simulink model "OpAmpCircuits2"  (R2021b)
settings: Solver=VariableStepAuto  StartTime=0.0  StopTime=inf  MaxStep=1e-5  RelTol=1e-3
libraries: fl_lib x55, nesl_utility x20, simulink x1
settings Model: PacingRate=0.010000  Creator=Work  LastModifiedBy=Work

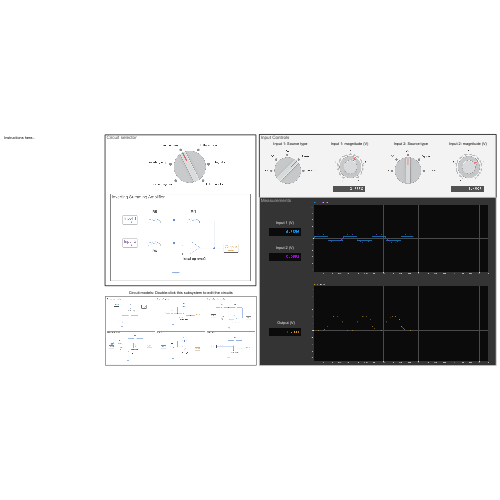
[thumbnail: Simulink's stored preview of the top-level diagram]
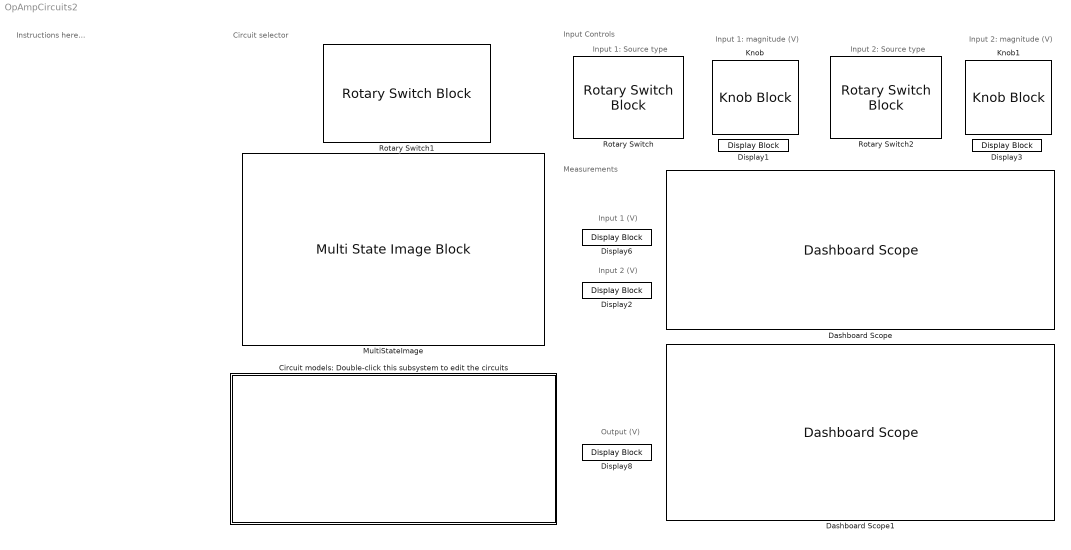
== system OpAmpCircuits2 ==
  note: Instructions here...
  note: Circuit selector
  note: Input 1: magnitude (V)
  note: Input 1: Source type
  note: Input Controls
  note: Measurements
  note: Input 1 (V)
  note: Output (V)
  note: Input 2 (V)
  note: Input 2: Source type
  note: Input 2: magnitude (V)
  Circuit models: Double-click this subsystem to edit the circuits : Subsystem
      mask Display: image('opampcircuits.png')
  Dashboard Scope : DashboardScope  TimeSpan=0.10000000000000001  Ymin=-11  Ymax=11  ScaleAtStop=off
  Dashboard Scope1 : DashboardScope  TimeSpan=0.10000000000000001  Ymin=-11  Ymax=11  ScaleAtStop=off
  Display{1..3,6,8} (5 alike) : DisplayBlock  LabelPosition=Hide  Format=Custom  Alignment=Right  Transparency=1  FormatString=%0.4f
  Knob : KnobBlock  LabelPosition=Hide  ScaleMin=-4  ScaleMax=4  TickInterval=2
  Knob1 : KnobBlock  LabelPosition=Hide  ScaleMin=-4  ScaleMax=4  TickInterval=2
  MultiStateImage : MultiStateImageBlock  LabelPosition=Hide
  Rotary Switch : RotarySwitchBlock  LabelPosition=Hide
      settings: Values={{'Off', 'DC', 'AC', 'Square', 'Triangle'}, [0 1 2 3 4]}
  Rotary Switch1 : RotarySwitchBlock  LabelPosition=Hide
      settings: Values={{'Noninverting amp', 'Inverting amp', 'Summing amp', 'Difference amp', 'Integrator', 'Differentiator'}, [1 2 3 4 5 6]}
  Rotary Switch2 : RotarySwitchBlock  LabelPosition=Hide
      settings: Values={{'Off', 'DC', 'AC', 'Square', 'Triangle'}, [0 1 2 3 4]}

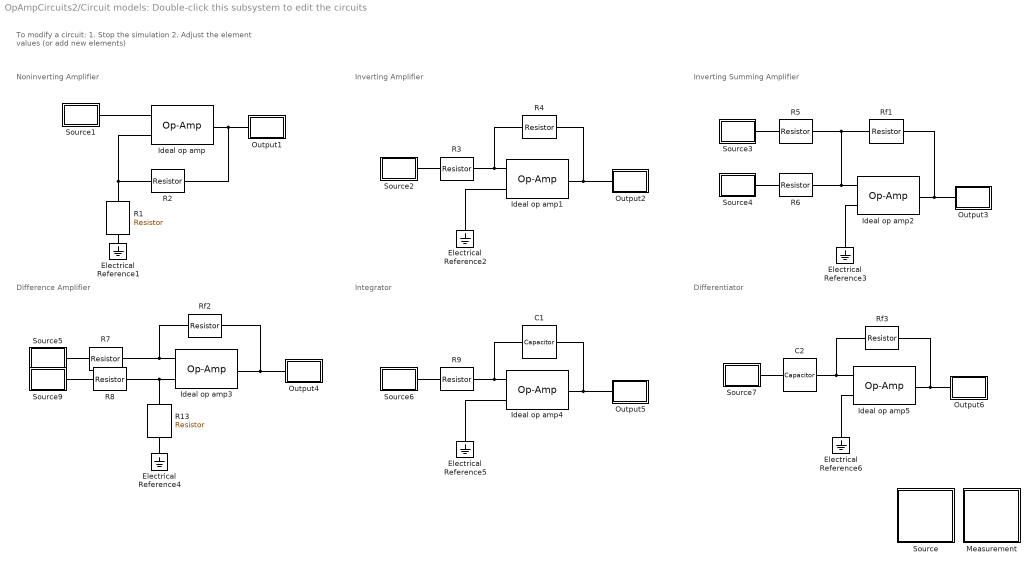
== system OpAmpCircuits2/Circuit models: Double-click this subsystem to edit the circuits ==
  note: To modify a circuit:
      |    1. Stop the simulation
      |    2. Adjust the element values (or add new elements)
  note: Differentiator
  note: Integrator
  note: Difference Amplifier
  note: Inverting Summing Amplifier
  note: Inverting Amplifier
  note: Noninverting Amplifier
  C1 : fl_lib/Electrical/Electrical Elements/Capacitor  c=1 uF  r=1e-6 Ohm  g=0 1/Ohm  i_specify=off  i_priority=None  i=0 A  i_nominal_specify=off  i_nominal_unit=A  i_nominal_value=1  v_specify=off  v_priority=None  v=0 V  v_nominal_specify=off  v_nominal_unit=V  v_nominal_value=1  vc_specify=off  vc_priority=High  vc=0 V  vc_nominal_specify=off  vc_nominal_unit=V  vc_nominal_value=1
      settings: AttributesFormatString=%<c> %<c_unit>
  C2 : fl_lib/Electrical/Electrical Elements/Capacitor  c=1 uF  r=1e-6 Ohm  g=0 1/Ohm  i_specify=off  i_priority=None  i=0 A  i_nominal_specify=off  i_nominal_unit=A  i_nominal_value=1  v_specify=off  v_priority=None  v=0 V  v_nominal_specify=off  v_nominal_unit=V  v_nominal_value=1  vc_specify=off  vc_priority=High  vc=0 V  vc_nominal_specify=off  vc_nominal_unit=V  vc_nominal_value=1
      settings: AttributesFormatString=%<c> %<c_unit>
  Electrical Reference{1..6} (6 alike) : fl_lib/Electrical/Electrical Elements/Electrical Reference
  Ideal op amp{,1..5} (6 alike) : fl_lib/Electrical/Electrical Elements/Op-Amp  outI_specify=off  outI_priority=None  outI=0 A  outI_nominal_specify=off  outI_nominal_unit=A  outI_nominal_value=1
  Measurement : Subsystem
  Output1 : Subsystem
      mask Display: image("output.png")
  Output2 : Subsystem
      mask Display: image("output.png")
  Output3 : Subsystem
      mask Display: image("output.png")
  Output4 : Subsystem
      mask Display: image("output.png")
  Output5 : Subsystem
      mask Display: image("output.png")
  Output6 : Subsystem
      mask Display: image("output.png")
  R{1..3,5..8,13} (8 alike) : fl_lib/Electrical/Electrical Elements/Resistor  R=1 kOhm  i_specify=off  i_priority=None  i=0 A  i_nominal_specify=off  i_nominal_unit=A  i_nominal_value=1  v_specify=off  v_priority=None  v=0 V  v_nominal_specify=off  v_nominal_unit=V  v_nominal_value=1
      settings: AttributesFormatString=%<R> %<R_unit>
  R4 : fl_lib/Electrical/Electrical Elements/Resistor  R=2 kOhm  i_specify=off  i_priority=None  i=0 A  i_nominal_specify=off  i_nominal_unit=A  i_nominal_value=1  v_specify=off  v_priority=None  v=0 V  v_nominal_specify=off  v_nominal_unit=V  v_nominal_value=1
      settings: AttributesFormatString=%<R> %<R_unit>
  R9 : fl_lib/Electrical/Electrical Elements/Resistor  R=2 kOhm  i_specify=off  i_priority=None  i=0 A  i_nominal_specify=off  i_nominal_unit=A  i_nominal_value=1  v_specify=off  v_priority=None  v=0 V  v_nominal_specify=off  v_nominal_unit=V  v_nominal_value=1
      settings: AttributesFormatString=%<R> %<R_unit>
  Rf1 : fl_lib/Electrical/Electrical Elements/Resistor  R=1 kOhm  i_specify=off  i_priority=None  i=0 A  i_nominal_specify=off  i_nominal_unit=A  i_nominal_value=1  v_specify=off  v_priority=None  v=0 V  v_nominal_specify=off  v_nominal_unit=V  v_nominal_value=1
      settings: AttributesFormatString=%<R> %<R_unit>
  Rf2 : fl_lib/Electrical/Electrical Elements/Resistor  R=1 kOhm  i_specify=off  i_priority=None  i=0 A  i_nominal_specify=off  i_nominal_unit=A  i_nominal_value=1  v_specify=off  v_priority=None  v=0 V  v_nominal_specify=off  v_nominal_unit=V  v_nominal_value=1
      settings: AttributesFormatString=%<R> %<R_unit>
  Rf3 : fl_lib/Electrical/Electrical Elements/Resistor  R=10 kOhm  i_specify=off  i_priority=None  i=0 A  i_nominal_specify=off  i_nominal_unit=A  i_nominal_value=1  v_specify=off  v_priority=None  v=0 V  v_nominal_specify=off  v_nominal_unit=V  v_nominal_value=1
      settings: AttributesFormatString=%<R> %<R_unit>
  Source : Subsystem
  Source1 : Subsystem
      mask Display: image("input1.png")
  Source2 : Subsystem
      mask Display: image("input1.png")
  Source3 : Subsystem
      mask Display: image("input1.png")
  Source4 : Subsystem
      mask Display: image("input2.png")
  Source5 : Subsystem
      mask Display: image("input1.png")
  Source6 : Subsystem
      mask Display: image("input1.png")
  Source7 : Subsystem
      mask Display: image("input1.png")
  Source9 : Subsystem
      mask Display: image("input2.png")
  connections:
  Ideal op amp5/LConn1 -- Electrical Reference6/LConn1
  Ideal op amp1/RConn1 -- Output2/LConn1 -- R4/LConn1
  R7/RConn1 -- Source5/RConn1
  C2/LConn1 -- Source7/RConn1
  Ideal op amp3/LConn2 -- Rf2/RConn1 -- R7/LConn1
  R8/RConn1 -- Source9/RConn1
  R6/RConn1 -- Source4/RConn1
  Source6/RConn1 -- R9/RConn1
  Ideal op amp4/RConn1 -- C1/RConn1 -- Output5/LConn1
  Output4/LConn1 -- Ideal op amp3/RConn1 -- Rf2/LConn1
  R2/RConn1 -- Ideal op amp/LConn2 -- R1/LConn1
  Ideal op amp/RConn1 -- Output1/LConn1 -- R2/LConn1
  Ideal op amp4/LConn1 -- Electrical Reference5/LConn1
  Source3/RConn1 -- R5/RConn1
  R13/RConn1 -- Electrical Reference4/LConn1
  Ideal op amp2/LConn1 -- Electrical Reference3/LConn1
  Ideal op amp5/LConn2 -- C2/RConn1 -- Rf3/RConn1
  Ideal op amp2/RConn1 -- Output3/LConn1 -- Rf1/LConn1
  Ideal op amp4/LConn2 -- C1/LConn1 -- R9/LConn1
  Ideal op amp1/LConn2 -- R3/LConn1 -- R4/RConn1
  Rf3/LConn1 -- Ideal op amp5/RConn1 -- Output6/LConn1
  Source2/RConn1 -- R3/RConn1
  R1/RConn1 -- Electrical Reference1/LConn1
  Ideal op amp1/LConn1 -- Electrical Reference2/LConn1
  Ideal op amp2/LConn2 -- R6/LConn1 -- R5/LConn1 -- Rf1/RConn1
  R8/LConn1 -- R13/LConn1 -- Ideal op amp3/LConn1
  Ideal op amp/LConn1 -- Source1/RConn1

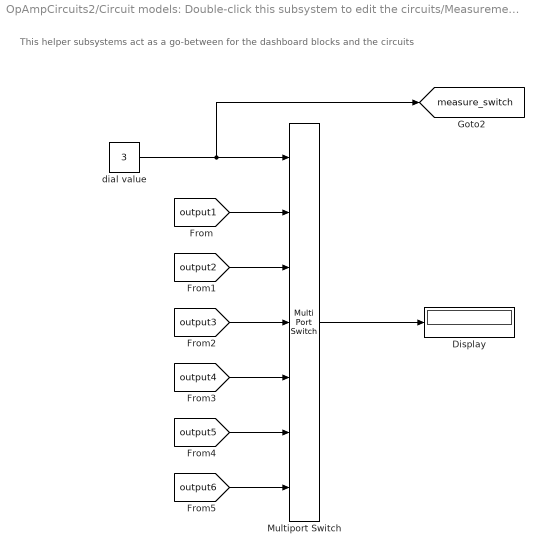
== system OpAmpCircuits2/Circuit models: Double-click this subsystem to edit the circuits/Measurement ==
  note: This helper subsystems act as a go-between for the dashboard blocks and the circuits
  Display : Display
  Multiport Switch : MultiPortSwitch  Inputs=6
  dial value : Constant  Value=3
  tag scope: measure_switch=global
  wires:
  [output1] -> Multiport Switch/2
  [output2] -> Multiport Switch/3
  [output3] -> Multiport Switch/4
  Multiport Switch/1 -> Display/1
  [output4] -> Multiport Switch/5
  [output5] -> Multiport Switch/6
  [output6] -> Multiport Switch/7
  dial value/1 -> [measure_switch], Multiport Switch/1

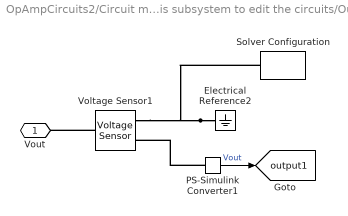
== system OpAmpCircuits2/Circuit models: Double-click this subsystem to edit the circuits/Output1 ==
  Electrical Reference2 : fl_lib/Electrical/Electrical Elements/Electrical Reference
  PS-Simulink Converter1 : nesl_utility/PS-Simulink Converter  PhysicalDomain=network_engine_domain  SubClassName=ps_output  LeftPortType=input  RightPortType=output  PseudoPeriodic=off  Frequencies=[]  Unit=inherit  AffineConversion=off
      settings: SourceProductBaseCode=PW,SS
  Solver Configuration : nesl_utility/Solver Configuration  PhysicalDomain=network_engine_domain  SubClassName=solver  LeftPortType=input  RightPortType=generic  Tones=[]  Harmonics=[]  SimulateNoise=off  Profile=off  UseLocalSampling=off  EnableSwitchedLinearOptims=on  FrequencyDomain=off  UseCCode=off  RelTol=0.001  AbsTol=1e-06  MinStep=1e-09  ToWorkspace=off  RevertToSquareIcSolve=off  NumHomotopyIterations=100  PhasorMode=off  PhasorModeNumHarmonics=1  DoDC=off  ResidualTolerance=1e-09  UseLocalSolver=off  LocalSolverChoice=NE_BACKWARD_EULER_ADVANCER  LocalSolverSampleTime=0.001  DoFixedCost=off  MaxNonlinIter=3  MaxModeIter=2  ComputeImpulses=off  ImpulseIterations=2  LinearAlgebra=auto  EquationFormulation=NE_TIME_EF  DelaysMemoryBudget=1024  AutomaticFiltering=on  FilteringTimeConstant=0.001  PartitionStorageMethod=AS_NEEDED  PartitionMemoryBudget=1024  PartitionMethod=ROBUST
      settings: SourceProductBaseCode=PW,SS
  Voltage Sensor1 : fl_lib/Electrical/Electrical Sensors/Voltage Sensor
  Vout : PMIOPort  Side=Left
  tag scope: output1=global
  wires:
  PS-Simulink Converter1/1 -> [output1]  "Vout"
  connections:
  Voltage Sensor1/LConn1 -- Vout/RConn1
  Electrical Reference2/LConn1 -- Voltage Sensor1/RConn2 -- Solver Configuration/RConn1
  PS-Simulink Converter1/LConn1 -- Voltage Sensor1/RConn1

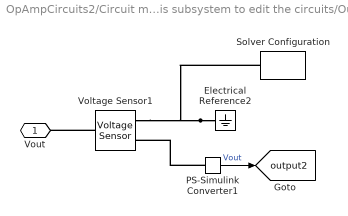
== system OpAmpCircuits2/Circuit models: Double-click this subsystem to edit the circuits/Output2 ==
  Electrical Reference2 : fl_lib/Electrical/Electrical Elements/Electrical Reference
  PS-Simulink Converter1 : nesl_utility/PS-Simulink Converter  PhysicalDomain=network_engine_domain  SubClassName=ps_output  LeftPortType=input  RightPortType=output  PseudoPeriodic=off  Frequencies=[]  Unit=inherit  AffineConversion=off
      settings: SourceProductBaseCode=PW,SS
  Solver Configuration : nesl_utility/Solver Configuration  PhysicalDomain=network_engine_domain  SubClassName=solver  LeftPortType=input  RightPortType=generic  Tones=[]  Harmonics=[]  SimulateNoise=off  Profile=off  UseLocalSampling=off  EnableSwitchedLinearOptims=on  FrequencyDomain=off  UseCCode=off  RelTol=0.001  AbsTol=1e-06  MinStep=1e-09  ToWorkspace=off  RevertToSquareIcSolve=off  NumHomotopyIterations=100  PhasorMode=off  PhasorModeNumHarmonics=1  DoDC=off  ResidualTolerance=1e-09  UseLocalSolver=off  LocalSolverChoice=NE_BACKWARD_EULER_ADVANCER  LocalSolverSampleTime=0.001  DoFixedCost=off  MaxNonlinIter=3  MaxModeIter=2  ComputeImpulses=off  ImpulseIterations=2  LinearAlgebra=auto  EquationFormulation=NE_TIME_EF  DelaysMemoryBudget=1024  AutomaticFiltering=on  FilteringTimeConstant=0.001  PartitionStorageMethod=AS_NEEDED  PartitionMemoryBudget=1024  PartitionMethod=ROBUST
      settings: SourceProductBaseCode=PW,SS
  Voltage Sensor1 : fl_lib/Electrical/Electrical Sensors/Voltage Sensor
  Vout : PMIOPort  Side=Left
  tag scope: output2=global
  wires:
  PS-Simulink Converter1/1 -> [output2]  "Vout"
  connections:
  Voltage Sensor1/LConn1 -- Vout/RConn1
  Electrical Reference2/LConn1 -- Voltage Sensor1/RConn2 -- Solver Configuration/RConn1
  PS-Simulink Converter1/LConn1 -- Voltage Sensor1/RConn1

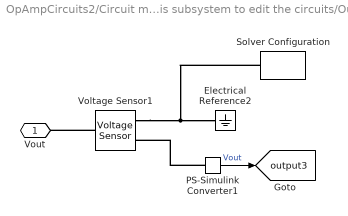
== system OpAmpCircuits2/Circuit models: Double-click this subsystem to edit the circuits/Output3 ==
  Electrical Reference2 : fl_lib/Electrical/Electrical Elements/Electrical Reference
  PS-Simulink Converter1 : nesl_utility/PS-Simulink Converter  PhysicalDomain=network_engine_domain  SubClassName=ps_output  LeftPortType=input  RightPortType=output  PseudoPeriodic=off  Frequencies=[]  Unit=inherit  AffineConversion=off
      settings: SourceProductBaseCode=PW,SS
  Solver Configuration : nesl_utility/Solver Configuration  PhysicalDomain=network_engine_domain  SubClassName=solver  LeftPortType=input  RightPortType=generic  Tones=[]  Harmonics=[]  SimulateNoise=off  Profile=off  UseLocalSampling=off  EnableSwitchedLinearOptims=on  FrequencyDomain=off  UseCCode=off  RelTol=0.001  AbsTol=1e-06  MinStep=1e-09  ToWorkspace=off  RevertToSquareIcSolve=off  NumHomotopyIterations=100  PhasorMode=off  PhasorModeNumHarmonics=1  DoDC=off  ResidualTolerance=1e-09  UseLocalSolver=off  LocalSolverChoice=NE_BACKWARD_EULER_ADVANCER  LocalSolverSampleTime=0.001  DoFixedCost=off  MaxNonlinIter=3  MaxModeIter=2  ComputeImpulses=off  ImpulseIterations=2  LinearAlgebra=auto  EquationFormulation=NE_TIME_EF  DelaysMemoryBudget=1024  AutomaticFiltering=on  FilteringTimeConstant=0.001  PartitionStorageMethod=AS_NEEDED  PartitionMemoryBudget=1024  PartitionMethod=ROBUST
      settings: SourceProductBaseCode=PW,SS
  Voltage Sensor1 : fl_lib/Electrical/Electrical Sensors/Voltage Sensor
  Vout : PMIOPort  Side=Left
  tag scope: output3=global
  wires:
  PS-Simulink Converter1/1 -> [output3]  "Vout"
  connections:
  Voltage Sensor1/LConn1 -- Vout/RConn1
  Voltage Sensor1/RConn2 -- Solver Configuration/RConn1 -- Electrical Reference2/LConn1
  PS-Simulink Converter1/LConn1 -- Voltage Sensor1/RConn1

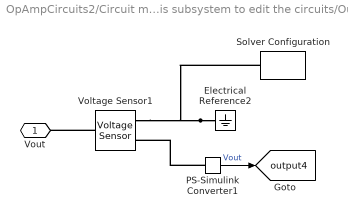
== system OpAmpCircuits2/Circuit models: Double-click this subsystem to edit the circuits/Output4 ==
  Electrical Reference2 : fl_lib/Electrical/Electrical Elements/Electrical Reference
  PS-Simulink Converter1 : nesl_utility/PS-Simulink Converter  PhysicalDomain=network_engine_domain  SubClassName=ps_output  LeftPortType=input  RightPortType=output  PseudoPeriodic=off  Frequencies=[]  Unit=inherit  AffineConversion=off
      settings: SourceProductBaseCode=PW,SS
  Solver Configuration : nesl_utility/Solver Configuration  PhysicalDomain=network_engine_domain  SubClassName=solver  LeftPortType=input  RightPortType=generic  Tones=[]  Harmonics=[]  SimulateNoise=off  Profile=off  UseLocalSampling=off  EnableSwitchedLinearOptims=on  FrequencyDomain=off  UseCCode=off  RelTol=0.001  AbsTol=1e-06  MinStep=1e-09  ToWorkspace=off  RevertToSquareIcSolve=off  NumHomotopyIterations=100  PhasorMode=off  PhasorModeNumHarmonics=1  DoDC=off  ResidualTolerance=1e-09  UseLocalSolver=off  LocalSolverChoice=NE_BACKWARD_EULER_ADVANCER  LocalSolverSampleTime=0.001  DoFixedCost=off  MaxNonlinIter=3  MaxModeIter=2  ComputeImpulses=off  ImpulseIterations=2  LinearAlgebra=auto  EquationFormulation=NE_TIME_EF  DelaysMemoryBudget=1024  AutomaticFiltering=on  FilteringTimeConstant=0.001  PartitionStorageMethod=AS_NEEDED  PartitionMemoryBudget=1024  PartitionMethod=ROBUST
      settings: SourceProductBaseCode=PW,SS
  Voltage Sensor1 : fl_lib/Electrical/Electrical Sensors/Voltage Sensor
  Vout : PMIOPort  Side=Left
  tag scope: output4=global
  wires:
  PS-Simulink Converter1/1 -> [output4]  "Vout"
  connections:
  Voltage Sensor1/LConn1 -- Vout/RConn1
  Electrical Reference2/LConn1 -- Voltage Sensor1/RConn2 -- Solver Configuration/RConn1
  PS-Simulink Converter1/LConn1 -- Voltage Sensor1/RConn1

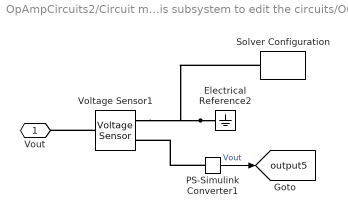
== system OpAmpCircuits2/Circuit models: Double-click this subsystem to edit the circuits/Output5 ==
  Electrical Reference2 : fl_lib/Electrical/Electrical Elements/Electrical Reference
  PS-Simulink Converter1 : nesl_utility/PS-Simulink Converter  PhysicalDomain=network_engine_domain  SubClassName=ps_output  LeftPortType=input  RightPortType=output  PseudoPeriodic=off  Frequencies=[]  Unit=inherit  AffineConversion=off
      settings: SourceProductBaseCode=PW,SS
  Solver Configuration : nesl_utility/Solver Configuration  PhysicalDomain=network_engine_domain  SubClassName=solver  LeftPortType=input  RightPortType=generic  Tones=[]  Harmonics=[]  SimulateNoise=off  Profile=off  UseLocalSampling=off  EnableSwitchedLinearOptims=on  FrequencyDomain=off  UseCCode=off  RelTol=0.001  AbsTol=1e-06  MinStep=1e-09  ToWorkspace=off  RevertToSquareIcSolve=off  NumHomotopyIterations=100  PhasorMode=off  PhasorModeNumHarmonics=1  DoDC=off  ResidualTolerance=1e-09  UseLocalSolver=off  LocalSolverChoice=NE_BACKWARD_EULER_ADVANCER  LocalSolverSampleTime=0.001  DoFixedCost=off  MaxNonlinIter=3  MaxModeIter=2  ComputeImpulses=off  ImpulseIterations=2  LinearAlgebra=auto  EquationFormulation=NE_TIME_EF  DelaysMemoryBudget=1024  AutomaticFiltering=on  FilteringTimeConstant=0.001  PartitionStorageMethod=AS_NEEDED  PartitionMemoryBudget=1024  PartitionMethod=ROBUST
      settings: SourceProductBaseCode=PW,SS
  Voltage Sensor1 : fl_lib/Electrical/Electrical Sensors/Voltage Sensor
  Vout : PMIOPort  Side=Left
  tag scope: output5=global
  wires:
  PS-Simulink Converter1/1 -> [output5]  "Vout"
  connections:
  Voltage Sensor1/LConn1 -- Vout/RConn1
  Electrical Reference2/LConn1 -- Voltage Sensor1/RConn2 -- Solver Configuration/RConn1
  PS-Simulink Converter1/LConn1 -- Voltage Sensor1/RConn1

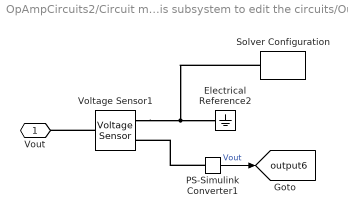
== system OpAmpCircuits2/Circuit models: Double-click this subsystem to edit the circuits/Output6 ==
  Electrical Reference2 : fl_lib/Electrical/Electrical Elements/Electrical Reference
  PS-Simulink Converter1 : nesl_utility/PS-Simulink Converter  PhysicalDomain=network_engine_domain  SubClassName=ps_output  LeftPortType=input  RightPortType=output  PseudoPeriodic=off  Frequencies=[]  Unit=inherit  AffineConversion=off
      settings: SourceProductBaseCode=PW,SS
  Solver Configuration : nesl_utility/Solver Configuration  PhysicalDomain=network_engine_domain  SubClassName=solver  LeftPortType=input  RightPortType=generic  Tones=[]  Harmonics=[]  SimulateNoise=off  Profile=off  UseLocalSampling=off  EnableSwitchedLinearOptims=on  FrequencyDomain=off  UseCCode=off  RelTol=0.001  AbsTol=1e-06  MinStep=1e-09  ToWorkspace=off  RevertToSquareIcSolve=off  NumHomotopyIterations=100  PhasorMode=off  PhasorModeNumHarmonics=1  DoDC=off  ResidualTolerance=1e-09  UseLocalSolver=off  LocalSolverChoice=NE_BACKWARD_EULER_ADVANCER  LocalSolverSampleTime=0.001  DoFixedCost=off  MaxNonlinIter=3  MaxModeIter=2  ComputeImpulses=off  ImpulseIterations=2  LinearAlgebra=auto  EquationFormulation=NE_TIME_EF  DelaysMemoryBudget=1024  AutomaticFiltering=on  FilteringTimeConstant=0.001  PartitionStorageMethod=AS_NEEDED  PartitionMemoryBudget=1024  PartitionMethod=ROBUST
      settings: SourceProductBaseCode=PW,SS
  Voltage Sensor1 : fl_lib/Electrical/Electrical Sensors/Voltage Sensor
  Vout : PMIOPort  Side=Left
  tag scope: output6=global
  wires:
  PS-Simulink Converter1/1 -> [output6]  "Vout"
  connections:
  Voltage Sensor1/LConn1 -- Vout/RConn1
  Voltage Sensor1/RConn2 -- Solver Configuration/RConn1 -- Electrical Reference2/LConn1
  PS-Simulink Converter1/LConn1 -- Voltage Sensor1/RConn1

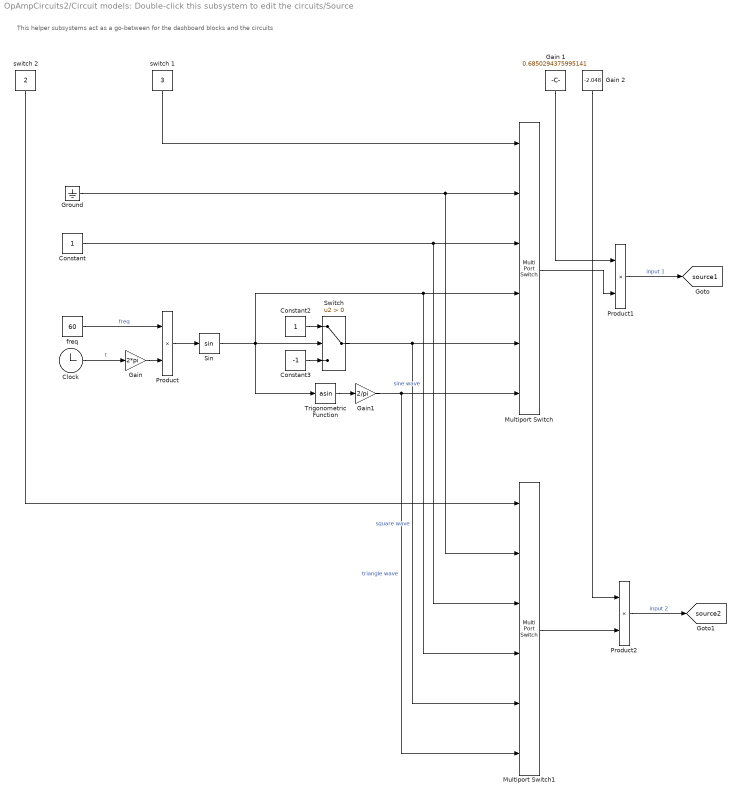
== system OpAmpCircuits2/Circuit models: Double-click this subsystem to edit the circuits/Source ==
  note: This helper subsystems act as a go-between for the dashboard blocks and the circuits
  Clock : Clock
  Constant : Constant
  Constant2 : Constant  SampleTime=0
  Constant3 : Constant  Value=-1  SampleTime=0
  Gain : Gain  Gain=2*pi
  Gain 1 : Constant  Value=0.6850294375995141
  Gain 2 : Constant  Value=-2.048
  Gain1 : Gain  Gain=2/pi
  Ground : Ground
  Multiport Switch : MultiPortSwitch  DataPortOrder=Zero-based contiguous  Inputs=5  zeroidx=on
  Multiport Switch1 : MultiPortSwitch  DataPortOrder=Zero-based contiguous  Inputs=5  zeroidx=on
  Product : Product
  Product1 : Product
  Product2 : Product
  Sin : Trigonometry
  Switch : Switch  Criteria=u2 > Threshold
  Trigonometric Function : Trigonometry  Operator=asin
  freq : Constant  Value=60  SampleTime=0
  switch 1 : Constant  Value=3
  switch 2 : Constant  Value=2
  tag scope: source1=global, source2=global
  wires:
  Multiport Switch/1 -> Product1/2
  switch 1/1 -> Multiport Switch/1
  switch 2/1 -> Multiport Switch1/1
  Gain1/1 -> Multiport Switch/6, Multiport Switch1/6  "triangle wave"
  Constant2/1 -> Switch/1
  Constant3/1 -> Switch/3
  Switch/1 -> Multiport Switch/5, Multiport Switch1/5  "square wave"
  Gain/1 -> Product/2
  Constant/1 -> Multiport Switch/3, Multiport Switch1/3
  Sin/1 -> Multiport Switch/4, Multiport Switch1/4, Trigonometric Function/1, Switch/2  "sine wave"
  Clock/1 -> Gain/1  "t"
  Trigonometric Function/1 -> Gain1/1
  freq/1 -> Product/1  "freq"
  Product/1 -> Sin/1
  Product1/1 -> [source1]  "input 1"
  Product2/1 -> [source2]  "input 2"
  Gain 1/1 -> Product1/1
  Multiport Switch1/1 -> Product2/2
  Gain 2/1 -> Product2/1
  Ground/1 -> Multiport Switch/2, Multiport Switch1/2

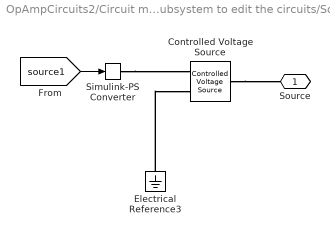
== system OpAmpCircuits2/Circuit models: Double-click this subsystem to edit the circuits/Source1 ==
  Controlled Voltage Source : fl_lib/Electrical/Electrical Sources/Controlled Voltage Source
  Electrical Reference3 : fl_lib/Electrical/Electrical Elements/Electrical Reference
  Simulink-PS Converter : nesl_utility/Simulink-PS Converter  PhysicalDomain=network_engine_domain  SubClassName=ps_input  LeftPortType=input  RightPortType=output  PseudoPeriodic=off  Frequencies=[]  NoiseDistribution=none  NoiseParameters=[]  Unit=1  AffineConversion=off  FilteringAndDerivatives=provide  SimscapeFilterOrder=1  InputFilterTimeConstant=0.001  UdotUserProvided=0
      settings: SourceProductBaseCode=PW,SS
  Source : PMIOPort  Side=Right
  wires:
  [source1] -> Simulink-PS Converter/1
  connections:
  Electrical Reference3/LConn1 -- Controlled Voltage Source/RConn2
  Controlled Voltage Source/LConn1 -- Source/RConn1
  Simulink-PS Converter/RConn1 -- Controlled Voltage Source/RConn1

== system OpAmpCircuits2/Circuit models: Double-click this subsystem to edit the circuits/Source2 ==
  Controlled Voltage Source : fl_lib/Electrical/Electrical Sources/Controlled Voltage Source
  Electrical Reference3 : fl_lib/Electrical/Electrical Elements/Electrical Reference
  Simulink-PS Converter : nesl_utility/Simulink-PS Converter  PhysicalDomain=network_engine_domain  SubClassName=ps_input  LeftPortType=input  RightPortType=output  PseudoPeriodic=off  Frequencies=[]  NoiseDistribution=none  NoiseParameters=[]  Unit=1  AffineConversion=off  FilteringAndDerivatives=provide  SimscapeFilterOrder=1  InputFilterTimeConstant=0.001  UdotUserProvided=0
      settings: SourceProductBaseCode=PW,SS
  Source : PMIOPort  Side=Right
  wires:
  [source1] -> Simulink-PS Converter/1
  connections:
  Electrical Reference3/LConn1 -- Controlled Voltage Source/RConn2
  Controlled Voltage Source/LConn1 -- Source/RConn1
  Simulink-PS Converter/RConn1 -- Controlled Voltage Source/RConn1

== system OpAmpCircuits2/Circuit models: Double-click this subsystem to edit the circuits/Source3 ==
  Controlled Voltage Source : fl_lib/Electrical/Electrical Sources/Controlled Voltage Source
  Electrical Reference3 : fl_lib/Electrical/Electrical Elements/Electrical Reference
  Simulink-PS Converter : nesl_utility/Simulink-PS Converter  PhysicalDomain=network_engine_domain  SubClassName=ps_input  LeftPortType=input  RightPortType=output  PseudoPeriodic=off  Frequencies=[]  NoiseDistribution=none  NoiseParameters=[]  Unit=1  AffineConversion=off  FilteringAndDerivatives=provide  SimscapeFilterOrder=1  InputFilterTimeConstant=0.001  UdotUserProvided=0
      settings: SourceProductBaseCode=PW,SS
  Source : PMIOPort  Side=Right
  wires:
  [source1] -> Simulink-PS Converter/1
  connections:
  Electrical Reference3/LConn1 -- Controlled Voltage Source/RConn2
  Controlled Voltage Source/LConn1 -- Source/RConn1
  Simulink-PS Converter/RConn1 -- Controlled Voltage Source/RConn1

== system OpAmpCircuits2/Circuit models: Double-click this subsystem to edit the circuits/Source4 ==
  Controlled Voltage Source : fl_lib/Electrical/Electrical Sources/Controlled Voltage Source
  Electrical Reference3 : fl_lib/Electrical/Electrical Elements/Electrical Reference
  Simulink-PS Converter : nesl_utility/Simulink-PS Converter  PhysicalDomain=network_engine_domain  SubClassName=ps_input  LeftPortType=input  RightPortType=output  PseudoPeriodic=off  Frequencies=[]  NoiseDistribution=none  NoiseParameters=[]  Unit=1  AffineConversion=off  FilteringAndDerivatives=provide  SimscapeFilterOrder=1  InputFilterTimeConstant=0.001  UdotUserProvided=0
      settings: SourceProductBaseCode=PW,SS
  Source : PMIOPort  Side=Right
  wires:
  [source2] -> Simulink-PS Converter/1
  connections:
  Electrical Reference3/LConn1 -- Controlled Voltage Source/RConn2
  Controlled Voltage Source/LConn1 -- Source/RConn1
  Simulink-PS Converter/RConn1 -- Controlled Voltage Source/RConn1

== system OpAmpCircuits2/Circuit models: Double-click this subsystem to edit the circuits/Source5 ==
  Controlled Voltage Source : fl_lib/Electrical/Electrical Sources/Controlled Voltage Source
  Electrical Reference3 : fl_lib/Electrical/Electrical Elements/Electrical Reference
  Simulink-PS Converter : nesl_utility/Simulink-PS Converter  PhysicalDomain=network_engine_domain  SubClassName=ps_input  LeftPortType=input  RightPortType=output  PseudoPeriodic=off  Frequencies=[]  NoiseDistribution=none  NoiseParameters=[]  Unit=1  AffineConversion=off  FilteringAndDerivatives=provide  SimscapeFilterOrder=1  InputFilterTimeConstant=0.001  UdotUserProvided=0
      settings: SourceProductBaseCode=PW,SS
  Source : PMIOPort  Side=Right
  wires:
  [source1] -> Simulink-PS Converter/1
  connections:
  Electrical Reference3/LConn1 -- Controlled Voltage Source/RConn2
  Controlled Voltage Source/LConn1 -- Source/RConn1
  Simulink-PS Converter/RConn1 -- Controlled Voltage Source/RConn1

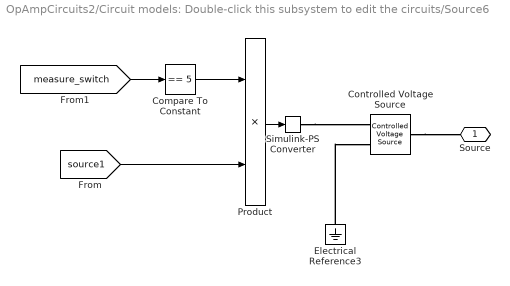
== system OpAmpCircuits2/Circuit models: Double-click this subsystem to edit the circuits/Source6 ==
  Compare To Constant : simulink/Logic and Bit Operations/Compare To Constant  relop===  const=5  OutDataTypeStr=boolean
  Controlled Voltage Source : fl_lib/Electrical/Electrical Sources/Controlled Voltage Source
  Electrical Reference3 : fl_lib/Electrical/Electrical Elements/Electrical Reference
  Product : Product
  Simulink-PS Converter : nesl_utility/Simulink-PS Converter  PhysicalDomain=network_engine_domain  SubClassName=ps_input  LeftPortType=input  RightPortType=output  PseudoPeriodic=off  Frequencies=[]  NoiseDistribution=none  NoiseParameters=[]  Unit=1  AffineConversion=off  FilteringAndDerivatives=provide  SimscapeFilterOrder=1  InputFilterTimeConstant=0.001  UdotUserProvided=0
      settings: SourceProductBaseCode=PW,SS
  Source : PMIOPort  Side=Right
  wires:
  [measure_switch] -> Compare To Constant/1
  Compare To Constant/1 -> Product/1
  Product/1 -> Simulink-PS Converter/1
  [source1] -> Product/2
  connections:
  Electrical Reference3/LConn1 -- Controlled Voltage Source/RConn2
  Controlled Voltage Source/LConn1 -- Source/RConn1
  Simulink-PS Converter/RConn1 -- Controlled Voltage Source/RConn1

== system OpAmpCircuits2/Circuit models: Double-click this subsystem to edit the circuits/Source7 ==
  Controlled Voltage Source : fl_lib/Electrical/Electrical Sources/Controlled Voltage Source
  Electrical Reference3 : fl_lib/Electrical/Electrical Elements/Electrical Reference
  Simulink-PS Converter : nesl_utility/Simulink-PS Converter  PhysicalDomain=network_engine_domain  SubClassName=ps_input  LeftPortType=input  RightPortType=output  PseudoPeriodic=off  Frequencies=[]  NoiseDistribution=none  NoiseParameters=[]  Unit=1  AffineConversion=off  FilteringAndDerivatives=provide  SimscapeFilterOrder=1  InputFilterTimeConstant=0.001  UdotUserProvided=0
      settings: SourceProductBaseCode=PW,SS
  Source : PMIOPort  Side=Right
  wires:
  [source1] -> Simulink-PS Converter/1
  connections:
  Electrical Reference3/LConn1 -- Controlled Voltage Source/RConn2
  Controlled Voltage Source/LConn1 -- Source/RConn1
  Simulink-PS Converter/RConn1 -- Controlled Voltage Source/RConn1

== system OpAmpCircuits2/Circuit models: Double-click this subsystem to edit the circuits/Source9 ==
  Controlled Voltage Source : fl_lib/Electrical/Electrical Sources/Controlled Voltage Source
  Electrical Reference3 : fl_lib/Electrical/Electrical Elements/Electrical Reference
  Simulink-PS Converter : nesl_utility/Simulink-PS Converter  PhysicalDomain=network_engine_domain  SubClassName=ps_input  LeftPortType=input  RightPortType=output  PseudoPeriodic=off  Frequencies=[]  NoiseDistribution=none  NoiseParameters=[]  Unit=1  AffineConversion=off  FilteringAndDerivatives=provide  SimscapeFilterOrder=1  InputFilterTimeConstant=0.001  UdotUserProvided=0
      settings: SourceProductBaseCode=PW,SS
  Source : PMIOPort  Side=Right
  wires:
  [source2] -> Simulink-PS Converter/1
  connections:
  Electrical Reference3/LConn1 -- Controlled Voltage Source/RConn2
  Controlled Voltage Source/LConn1 -- Source/RConn1
  Simulink-PS Converter/RConn1 -- Controlled Voltage Source/RConn1
